simulink model "irep_force_control_simu"  (Simulink 8.5)
settings: Solver=ode3  StartTime=0.0  StopTime=inf  FixedStep=dt  RelTol=1e-3
InitFcn:
  | IREP_DEPENDENCY
  | init_omni
  | init_filters
  | init_invivo
  | init_telemanipulation
  | init_parker_xyz
  | init_magnetic_tracker
  | init_loadcell
  | init_scopes
  | init_homing
  | init_force_control
  | init_xpc_invivo_simu
undefined symbols (not defined in the file): ang_vel_scale, B_simu, beta, camera_home_voltage, counter_offset, dt, dt_trakstar, E_Y, encoder_counts, epsilon_robust_inverse, gear_ratio, HomingFineEps, HomingRoughEps, HomingRoughVelocity, I1_primary, I1_secondary, I2_primary, I2_secondary, irep_parameters_left, irep_parameters_right, joystick_filter_coeffs, K_d, K_i, K_naive_inv, K_p, k_right, L1l, L1r, L2l, L2r, L_zeus, left_arm_home_voltage, left_x0_parallelogram, LeftArmHomingDirectionVector, LeftArmHomingIntGain, lin_vel_scale, LOADCELL_BIAS, LOADCELL_GAIN, max_conf_space_speed, N_joystick, N_pots, N_trakstar, OmegaMax, OmegaMin, orientation_epsilon, position_epsilon, pots_filter_coeffs, q_eps_backlash, quadrature_mode, r, right_arm_home_voltage, RightArmHomingDirectionVector, RightArmHomingIntGain, screw_pitch, statics_param, tau_compression_bias, tau_compression_gains, tau_neutral_deadband, tau_tension_bias, tau_tension_gains ... (+14)
libraries: slrtlib x38, xpcrtudplib x13, xpcobsoletelib x13, simulink x6, dspswit3 x2, dspsigops x1
(part 4 of 6)

== system irep_force_control_simu/Trajectory Planner/Left Arm/High Level/Actuation Compensation/Parallelogram Backlash  Compensatior ==
  q des : Inport
  Backlash Compensator : MATLAB Function  TreatAsAtomicUnit=on
  Bus Selector : BusSelector  OutputSignals=q2; q3
  Discrete Derivative : simulink/Discrete/Discrete Derivative  gainval=1.0  ICPrevScaledInput=0.0  InputProcessing=Inherited  OutMin=[]  OutMax=[]  OutDataType=fixdt(1, 16)  OutScaling=2^-10  DoSatur=off
  comp close : Constant  Value=0.5
  comp open : Constant  Value=-1
  epsilon : Outport
  wires:
  q des/1 -> Bus Selector/1
  Bus Selector/1 -> Discrete Derivative/1, Backlash Compensator/1(q_curr)  "<q2; q3>"
  Discrete Derivative/1 -> Backlash Compensator/2(q_dot_curr)  "q dot curr"
  Backlash Compensator/1(epsilon) -> epsilon/1
  comp open/1 -> Backlash Compensator/3(q2_comp_open)
  comp close/1 -> Backlash Compensator/4(q2_comp_close)

== system irep_force_control_simu/Trajectory Planner/Left Arm/High Level/Configuration Space/Parallelogram ==
  Enable : EnablePort
  5th Order Polynomial : Subsystem
  b_des : Constant  Value=[left_x0_parallelogram z0_parallelogram]  SampleTime=dt
  b1 : Outport
  wires:
  5th Order Polynomial/1(b) -> b1/1
  b_des/1 -> 5th Order Polynomial/1(b des)

== system irep_force_control_simu/Trajectory Planner/Left Arm/High Level/Configuration Space/Stem ==
  Enable : EnablePort
  5th Order Polynomial : Subsystem
  Terminator : Terminator
  enable : Constant  Value=0  SampleTime=dt
  psi des : Constant  Value=[pi/2;0;pi/2;0;0]  SampleTime=dt
  psi0 : Constant  Value=[pi/2;0;pi/2;0;0]  SampleTime=dt
  psi dot : Outport  InitialOutput=zeros(5,1)
  wires:
  enable/1 -> 5th Order Polynomial/3(enable)
  psi0/1 -> 5th Order Polynomial/2(psi0)
  psi des/1 -> 5th Order Polynomial/1(psi des)
  5th Order Polynomial/2(psi dot) -> psi dot/1
  5th Order Polynomial/1(psi) -> Terminator/1

== system irep_force_control_simu/Trajectory Planner/Left Arm/High Level/Inverse Istantaneous Kinematics/Coordination Module ==
  b1 : Inport
  q par : Inport  Port=2
  5-Bar Inverse Kinematics : MATLAB Function  TreatAsAtomicUnit=on
  Add : Sum  Inputs=+-  SampleTime=dt
  Coordination Block : MATLAB Function  TreatAsAtomicUnit=on
  L0 : Constant  Value=L_zeus  SampleTime=dt
  b0 : Constant  Value=[x0_parallelogram z0_parallelogram]  SampleTime=dt
  q1 : Outport
  "q2, q3" : Outport  Port=2
  wires:
  Add/1 -> "q2, q3"/1
  q par/1 -> Coordination Block/2(q_par)
  b1/1 -> Coordination Block/1(b1)
  Coordination Block/1(q1) -> q1/1
  5-Bar Inverse Kinematics/1(q) -> Add/2
  L0/1 -> Coordination Block/3(L0)
  b0/1 -> 5-Bar Inverse Kinematics/1(b1)
  Coordination Block/2(q23) -> Add/1

== system irep_force_control_simu/Trajectory Planner/Left Arm/High Level/Inverse Istantaneous Kinematics/Jaw Open/Close Module ==
  note: Temp fix,
      | teleop GP not working
  sensors : Inport
  Enable : EnablePort
  Bus Selector : BusSelector  OutputSignals=MSG_Type,gripper
  Jaw Open/Close : MATLAB Function  TreatAsAtomicUnit=on
  MTML_GP_max : Constant
  MTML_GP_min : Constant  Value=-1.3
  Unit Delay : UnitDelay  SampleTime=-1
  q9 : Outport
  wires:
  sensors/1 -> Bus Selector/1
  Jaw Open/Close/1(y) -> q9/1, Unit Delay/1
  MTML_GP_max/1 -> Jaw Open/Close/3(MTM_GP_max)
  MTML_GP_min/1 -> Jaw Open/Close/4(MTM_GP_min)
  Bus Selector/2 -> Jaw Open/Close/2(u)  "<gripper>"
  Bus Selector/1 -> Jaw Open/Close/1(MSG_valid)  "<MSG_Type>"
  Unit Delay/1 -> Jaw Open/Close/5(q9_prev)

== system irep_force_control_simu/Trajectory Planner/Left Arm/High Level/Task Space/Compute Weigths ==
  sensors : Inport
  conf space : Inport  Port=2
  Bus Selector : BusSelector  OutputSignals=b1 curr,psi curr
  Bus Selector1 : BusSelector  OutputSignals=foot switches
  joint limits : Constant  Value=[-x0_parallelogram_max -x0_parallelogram z0_parallelogram z0_parallelogram_max theta_min1 theta_max theta_min2 theta_max wrist_min wrist_max]  SampleTime=dt
  select weights : MATLAB Function  TreatAsAtomicUnit=on
  w min : Constant  Value=w_min  SampleTime=dt
  weights : Outport
  wires:
  joint limits/1 -> select weights/3(joint_limits)
  Bus Selector/1 -> select weights/1(b1)  "<b1 curr>"
  Bus Selector/2 -> select weights/2(psi)  "<psi curr>"
  conf space/1 -> Bus Selector/1
  select weights/1(W) -> weights/1
  w min/1 -> select weights/4(w_min)
  sensors/1 -> Bus Selector1/1
  Bus Selector1/1 -> select weights/5(foot_switches)  "<foot switches>"

== system irep_force_control_simu/Trajectory Planner/Left Arm/High Level/Task Space/Desired Twist Module ==
  note: Desired Twist Module v 1.1 - © 2011 Andrea Bajo, Nabil Simaan
  current pose : Inport
  des pose : Inport  Port=2
  Bus Selector1 : BusSelector  OutputSignals=p in world,R in world
  Bus Selector2 : BusSelector  OutputSignals=position,R,MSG_Type
  Compute Twist : MATLAB Function  TreatAsAtomicUnit=on
  Omega Max : Constant  Value=OmegaMax  SampleTime=dt
  Omega Min : Constant  Value=OmegaMin  SampleTime=dt
  Terminator : Terminator
  V Max : Constant  Value=Vmax  SampleTime=dt
  V Min : Constant  Value=Vmin  SampleTime=dt
  ang vel scale : Constant  Value=ang_vel_scale  SampleTime=dt
  lin vel scale : Constant  Value=lin_vel_scale  SampleTime=dt
  orientation epsilon : Constant  Value=orientation_epsilon  SampleTime=dt
  position epsilon : Constant  Value=position_epsilon  SampleTime=dt
  x des : Outport
  wires:
  Bus Selector1/1 -> Compute Twist/4(p_curr)  "<p in world>"
  Compute Twist/1(x_des) -> x des/1
  current pose/1 -> Bus Selector1/1
  Bus Selector1/2 -> Compute Twist/5(R_curr)  "<R in world>"
  Bus Selector2/1 -> Compute Twist/1(p_des)  "<position>"
  Bus Selector2/2 -> Compute Twist/2(R_des)  "<R>"
  des pose/1 -> Bus Selector2/1
  Bus Selector2/3 -> Compute Twist/3(MSG_Type)  "<MSG_Type>"
  V Max/1 -> Compute Twist/6(Vmax)
  Omega Max/1 -> Compute Twist/10(OmegaMax)
  V Min/1 -> Compute Twist/7(Vmin)
  Omega Min/1 -> Compute Twist/11(OmegaMin)
  position epsilon/1 -> Compute Twist/8(position_epsilon)
  orientation epsilon/1 -> Compute Twist/12(orientation_epsilon)
  lin vel scale/1 -> Compute Twist/9(lin_vel_scale)
  ang vel scale/1 -> Compute Twist/13(ang_vel_scale)
  Compute Twist/2(theta) -> Terminator/1

== system irep_force_control_simu/Trajectory Planner/Left Arm/High Level/Task Space/Direct Kinematics IREP ==
  "b1, psi" : Inport
  Bus Creator : BusCreator  Inputs=2
  Bus Selector : BusSelector  OutputSignals=Parker insertion stage,b1 curr,psi curr
  Direct Kinematic IREP : MATLAB Function  TreatAsAtomicUnit=on
  IREP parameters : Constant  Value=irep_parameters_left  SampleTime=dt
  Current Pose : Outport
  wires:
  "b1, psi"/1 -> Bus Selector/1
  Bus Selector/2 -> Direct Kinematic IREP/2(b1)  "<b1 curr>"
  Bus Selector/3 -> Direct Kinematic IREP/3(psi)  "<psi curr>"
  Direct Kinematic IREP/1(p) -> Bus Creator/1  "p in world"
  Direct Kinematic IREP/2(R) -> Bus Creator/2  "R in world"
  Bus Creator/1 -> Current Pose/1
  IREP parameters/1 -> Direct Kinematic IREP/4(parameters)
  Bus Selector/1 -> Direct Kinematic IREP/1(b0)  "<Parker insertion stage>"

== system irep_force_control_simu/Trajectory Planner/Left Arm/High Level/Task Space/Jxpsi Inverse IREP ==
  x des : Inport
  weights : Inport  Port=2
  "b1, psi" : Inport  Port=3
  Bus Selector1 : BusSelector  OutputSignals=Parker insertion stage,b1 curr,psi curr
  IREP parameters : Constant  Value=irep_parameters_left  SampleTime=dt
  Jxpsi Inverse IREP : MATLAB Function  TreatAsAtomicUnit=on
  epsilon : Constant  Value=epsilon_robust_inverse  SampleTime=dt
  max conf space speed : Constant  Value=max_conf_space_speed  SampleTime=dt
  conf dot des : Outport  PortDimensions=8
  wires:
  x des/1 -> Jxpsi Inverse IREP/1(x_des)
  Bus Selector1/3 -> Jxpsi Inverse IREP/4(psi)  "<psi curr>"
  Bus Selector1/2 -> Jxpsi Inverse IREP/3(b1)  "<b1 curr>"
  "b1, psi"/1 -> Bus Selector1/1
  Jxpsi Inverse IREP/1(conf_space_dot) -> conf dot des/1
  epsilon/1 -> Jxpsi Inverse IREP/7(epsilon_in)
  Bus Selector1/1 -> Jxpsi Inverse IREP/2(b0)  "<Parker insertion stage>"
  max conf space speed/1 -> Jxpsi Inverse IREP/8(max_ang_speed)
  weights/1 -> Jxpsi Inverse IREP/6(weights)
  IREP parameters/1 -> Jxpsi Inverse IREP/5(parameters)

== system irep_force_control_simu/Trajectory Planner/Left Arm/High Level/Task Space/Receive Desired Pose from MTM ==
  note: Telemanipulation Module v 1.0 - © COPYRIGHT 2010 Andrea Bajo, Nabil Simaan
  Master : Inport
  Bus Creator : BusCreator
  Bus Selector : BusSelector  OutputSignals=position,orientation (quat),MSG_Type,gripper
  Quaternion To Rotation : MATLAB Function  TreatAsAtomicUnit=on
  "pose, flags" : Outport
  wires:
  Bus Creator/1 -> "pose, flags"/1
  Master/1 -> Bus Selector/1
  Bus Selector/1 -> Bus Creator/1  "<position>"
  Quaternion To Rotation/1(R) -> Bus Creator/2
  Bus Selector/2 -> Quaternion To Rotation/1(quat)  "<orientation (quat)>"
  Bus Selector/3 -> Bus Creator/3  "<MSG_Type>"
  Bus Selector/4 -> Bus Creator/4  "<gripper>"

== system irep_force_control_simu/Trajectory Planner/Left Arm/High Level/Task Space/right task space scope ==
  In : Inport
  Bus Selector7 : BusSelector  OutputSignals=position,R,gripper,MSG_Type
  Gain : Gain
  Mux : Mux  Inputs=5
  R_to_axis_angle1 : MATLAB Function  TreatAsAtomicUnit=on
  left task space : slrtlib/Displays and Logging/Scope   scopeno=18  scopetype=Host  autostart=on  viewmode=Numerical  formatstr=scope_format_left_task_space_des  grid=on  ylimits=[0,0]  nosamples=10  noprepostsamples=0  interleave=1  triggermode=FreeRun  triggersignal=1  trigsignalfromport=off  triggerlevel=0.0  triggerslope=Either  triggerscope=1  triggersample=0  filename=weights1.dat  mode=Lazy  writesize=512  autorestart=off  dynamicfilemode=off  maxwritefilesize=512*1024^2
  wires:
  Mux/1 -> Gain/1
  In/1 -> Bus Selector7/1
  Bus Selector7/2 -> R_to_axis_angle1/1(R)  "<R>"
  Gain/1 -> left task space/1
  Bus Selector7/1 -> Mux/1  "<position>"
  R_to_axis_angle1/1(n_vec) -> Mux/2
  R_to_axis_angle1/2(theta) -> Mux/3
  Bus Selector7/3 -> Mux/4  "<gripper>"
  Bus Selector7/4 -> Mux/5  "<MSG_Type>"

== system irep_force_control_simu/Trajectory Planner/Left Arm/Low Level/Home Procedure/Fine Homing - Integral Control ==
  error : Inport
  Enable : EnablePort  StatesWhenEnabling=reset
  Discrete-Time Integrator : DiscreteIntegrator  SampleTime=dt  LimitOutput=on  UpperSaturationLimit=8  LowerSaturationLimit=-8
  Integral Gain : Gain  Gain=diag(LeftArmHomingIntGain)  Multiplication=Matrix(K*u)  SampleTime=dt
  q_des_fine : Outport  InitialOutput=zeros(9,1)
  wires:
  error/1 -> Integral Gain/1
  Discrete-Time Integrator/1 -> q_des_fine/1
  Integral Gain/1 -> Discrete-Time Integrator/1

== system irep_force_control_simu/Trajectory Planner/Left Arm/Low Level/Home Procedure/Homing Flags ==
  u : Inport
  Homing Completion : MATLAB Function  TreatAsAtomicUnit=on
  HomingFineEps : Constant  Value=HomingFineEps  SampleTime=dt
  Terminator1 : Terminator
  Unit Delay : UnitDelay  InitialCondition=zeros(9,1)  SampleTime=-1
  dt : Constant  Value=dt  SampleTime=dt
  wires:
  Homing Completion/1(Homed) -> Terminator1/1
  HomingFineEps/1 -> Homing Completion/2(EPS)
  u/1 -> Homing Completion/1(u)
  Homing Completion/2(Homed_T) -> Unit Delay/1
  Unit Delay/1 -> Homing Completion/4(Homed_T_prev)
  dt/1 -> Homing Completion/3(dt)

== system irep_force_control_simu/Trajectory Planner/Right Arm/High Level/Actuation Compensation/Compute Taus ==
  In1 : Inport
  In2 : Inport  Port=2
  Compute Tau : MATLAB Function  TreatAsAtomicUnit=on
  k_right : Constant  Value=k_right  SampleTime=dt
  tau : Outport
  wires:
  k_right/1 -> Compute Tau/3(k_right)
  In1/1 -> Compute Tau/1(GradU)
  Compute Tau/1(tau) -> tau/1
  In2/1 -> Compute Tau/2(conf_space)

== system irep_force_control_simu/Trajectory Planner/Right Arm/High Level/Actuation Compensation/Grad U1 ==
  conf space : Inport
  q : Inport  Port=2
  Compute grad U : MATLAB Function  TreatAsAtomicUnit=on
  Constant : Constant  Value=L1r  SampleTime=dt
  E_Y : Constant  Value=E_Y  SampleTime=dt
  Ip : Constant  Value=I1_primary+I2_primary  SampleTime=dt
  Is : Constant  Value=I1_secondary+I2_secondary  SampleTime=dt
  beta : Constant  Value=beta  SampleTime=dt
  r : Constant  Value=r  SampleTime=dt
  theta_0 : Constant  Value=theta0  SampleTime=dt
  grad_U : Outport
  wires:
  Constant/1 -> Compute grad U/3(L_p)
  beta/1 -> Compute grad U/9(beta)
  theta_0/1 -> Compute grad U/8(theta_0)
  r/1 -> Compute grad U/4(r)
  Ip/1 -> Compute grad U/6(Ip)
  E_Y/1 -> Compute grad U/5(E_Y)
  Compute grad U/1(grad_U) -> grad_U/1
  conf space/1 -> Compute grad U/1(conf_space)
  q/1 -> Compute grad U/2(q)
  Is/1 -> Compute grad U/7(Is)

== system irep_force_control_simu/Trajectory Planner/Right Arm/High Level/Actuation Compensation/Grad U2 ==
  conf space : Inport
  q : Inport  Port=2
  Compute grad U : MATLAB Function  TreatAsAtomicUnit=on
  Constant : Constant  Value=L2r  SampleTime=dt
  E_Y : Constant  Value=E_Y  SampleTime=dt
  Ip : Constant  Value=I2_primary  SampleTime=dt
  Is : Constant  Value=I2_secondary  SampleTime=dt
  beta : Constant  Value=beta  SampleTime=dt
  r : Constant  Value=r  SampleTime=dt
  theta_0 : Constant  Value=theta0  SampleTime=dt
  grad_U : Outport
  wires:
  Is/1 -> Compute grad U/7(Is)
  q/1 -> Compute grad U/2(q)
  conf space/1 -> Compute grad U/1(conf_space)
  Compute grad U/1(grad_U) -> grad_U/1
  E_Y/1 -> Compute grad U/5(E_Y)
  Ip/1 -> Compute grad U/6(Ip)
  r/1 -> Compute grad U/4(r)
  theta_0/1 -> Compute grad U/8(theta_0)
  beta/1 -> Compute grad U/9(beta)
  Constant/1 -> Compute grad U/3(L_p)

== system irep_force_control_simu/Trajectory Planner/Right Arm/High Level/Actuation Compensation/Parallelogram Backlash  Compensatior ==
  q des : Inport
  Backlash Compensator : MATLAB Function  TreatAsAtomicUnit=on
  Bus Selector : BusSelector  OutputSignals=q2;q3
  Discrete Derivative : simulink/Discrete/Discrete Derivative  gainval=1.0  ICPrevScaledInput=0.0  InputProcessing=Inherited  OutMin=[]  OutMax=[]  OutDataType=fixdt(1, 16)  OutScaling=2^-10  DoSatur=off
  comp close : Constant  Value=0
  comp close1 : Constant  Value=0.6
  comp open : Constant  Value=0
  comp open1 : Constant  Value=-1.2
  epsilon : Outport
  wires:
  q des/1 -> Bus Selector/1
  Bus Selector/1 -> Discrete Derivative/1, Backlash Compensator/1(q_curr)  "<q2;q3>"
  Discrete Derivative/1 -> Backlash Compensator/2(q_dot_curr)  "q dot curr"
  Backlash Compensator/1(epsilon) -> epsilon/1
  comp open/1 -> Backlash Compensator/3(q1_comp_open)
  comp close/1 -> Backlash Compensator/4(q1_comp_close)
  comp open1/1 -> Backlash Compensator/5(q2_comp_open)
  comp close1/1 -> Backlash Compensator/6(q2_comp_close)

== system irep_force_control_simu/Trajectory Planner/Right Arm/High Level/Actuation Compensation/get q_dot sign ==
  conf_space_dot : Inport
  conf_space : Inport  Port=2
  Dead Zone : DeadZone  LowerValue=-1e-3  UpperValue=1e-3  SaturateOnIntegerOverflow=on
  Unit Delay : UnitDelay  SampleTime=-1
  compute q_dot : MATLAB Function  TreatAsAtomicUnit=on
  q_dot_sign : MATLAB Function  TreatAsAtomicUnit=on
  q_dot_sgn : Outport
  wires:
  conf_space_dot/1 -> compute q_dot/2(conf_space_dot)
  conf_space/1 -> compute q_dot/1(conf_space)
  q_dot_sign/1(q_dot_sign_out) -> q_dot_sgn/1, Unit Delay/1
  Unit Delay/1 -> q_dot_sign/2(q_dot_sign_prev)
  compute q_dot/1(q_dot) -> Dead Zone/1
  Dead Zone/1 -> q_dot_sign/1(q_dot_sign_in)

== system irep_force_control_simu/Trajectory Planner/Right Arm/High Level/Actuation Compensation/q_eps 5th order poly ==
  q_eps_ref : Inport
  enable : Inport  Port=2
  Constant : Constant  Value=q_eps_backlash
  Digital Clock : DigitalClock  SampleTime=dt
  Embedded MATLAB Function : MATLAB Function  TreatAsAtomicUnit=on
  Terminator : Terminator
  Unit Delay : UnitDelay  SampleTime=dt
  Unit Delay1 : UnitDelay  SampleTime=dt
  Unit Delay2 : UnitDelay  InitialCondition=zeros(9,1)  SampleTime=dt
  tf : Constant  Value=5  SampleTime=dt
  q_eps_des : Outport
  wires:
  Embedded MATLAB Function/3(confn) -> Unit Delay/1
  Unit Delay/1 -> Embedded MATLAB Function/5(conf)
  Embedded MATLAB Function/4(t0n) -> Unit Delay1/1
  Embedded MATLAB Function/5(p0n) -> Unit Delay2/1
  Unit Delay2/1 -> Embedded MATLAB Function/7(p0)
  Unit Delay1/1 -> Embedded MATLAB Function/6(t0)
  Digital Clock/1 -> Embedded MATLAB Function/4(tc)
  q_eps_ref/1 -> Embedded MATLAB Function/1(p_des)
  Embedded MATLAB Function/1(p) -> q_eps_des/1
  tf/1 -> Embedded MATLAB Function/3(tf)
  enable/1 -> Embedded MATLAB Function/8(enable)
  Constant/1 -> Embedded MATLAB Function/2(p_curr)
  Embedded MATLAB Function/2(pdot) -> Terminator/1

== system irep_force_control_simu/Trajectory Planner/Right Arm/High Level/Configuration Space/Parallelogram ==
  Enable : EnablePort
  5th Order Polynomial : Subsystem
  b_des : Constant  Value=[x0_parallelogram z0_parallelogram]  SampleTime=dt
  b1 : Outport
  wires:
  b_des/1 -> 5th Order Polynomial/1(b des)
  5th Order Polynomial/1(b) -> b1/1

== system irep_force_control_simu/Trajectory Planner/Right Arm/High Level/Configuration Space/Stem ==
  Enable : EnablePort
  5th Order Polynomial : Subsystem
  Terminator : Terminator
  enable : Constant  Value=0  SampleTime=dt
  psi des : Constant  Value=[pi/2;0;pi/2;0;0]  SampleTime=dt
  psi0 : Constant  Value=[pi/2;0;pi/2;0;0]  SampleTime=dt
  psi dot : Outport  InitialOutput=zeros(5,1)
  wires:
  5th Order Polynomial/2(psi dot) -> psi dot/1
  psi des/1 -> 5th Order Polynomial/1(psi des)
  psi0/1 -> 5th Order Polynomial/2(psi0)
  enable/1 -> 5th Order Polynomial/3(enable)
  5th Order Polynomial/1(psi) -> Terminator/1

== system irep_force_control_simu/Trajectory Planner/Right Arm/High Level/Inverse Istantaneous Kinematics/Coordination Module ==
  b1 : Inport
  q par : Inport  Port=2
  5-Bar Inverse Kinematics : MATLAB Function  TreatAsAtomicUnit=on
  Add : Sum  Inputs=+-  SampleTime=dt
  Coordination Block : MATLAB Function  TreatAsAtomicUnit=on
  L0 : Constant  Value=L_zeus  SampleTime=dt
  b0 : Constant  Value=[x0_parallelogram z0_parallelogram]  SampleTime=dt
  q1 : Outport
  "q2, q3" : Outport  Port=2
  wires:
  Add/1 -> "q2, q3"/1
  q par/1 -> Coordination Block/2(q_par)
  b1/1 -> Coordination Block/1(b1)
  Coordination Block/1(q1) -> q1/1
  5-Bar Inverse Kinematics/1(q) -> Add/2
  L0/1 -> Coordination Block/3(L0)
  b0/1 -> 5-Bar Inverse Kinematics/1(b1)
  Coordination Block/2(q23) -> Add/1

== system irep_force_control_simu/Trajectory Planner/Right Arm/High Level/Inverse Istantaneous Kinematics/Jaw Open/Close Module ==
  sensors : Inport
  Enable : EnablePort
  Bus Selector : BusSelector  OutputSignals=MSG_Type,gripper
  Jaw Open/Close : MATLAB Function  TreatAsAtomicUnit=on
  MTM_GP_max : Constant  Value=1.05
  MTM_GP_min : Constant  Value=-0.48
  Unit Delay : UnitDelay  SampleTime=-1
  Unit Delay1 : UnitDelay  SampleTime=-1
  q9 : Outport
  wires:
  sensors/1 -> Bus Selector/1
  Jaw Open/Close/1(y) -> Unit Delay/1, Unit Delay1/1
  Bus Selector/2 -> Jaw Open/Close/2(u)  "<gripper>"
  MTM_GP_max/1 -> Jaw Open/Close/3(MTM_GP_max)
  MTM_GP_min/1 -> Jaw Open/Close/4(MTM_GP_min)
  Bus Selector/1 -> Jaw Open/Close/1(MSG_valid)  "<MSG_Type>"
  Unit Delay/1 -> Jaw Open/Close/5(q9_prev)
  Unit Delay1/1 -> q9/1

== system irep_force_control_simu/Trajectory Planner/Right Arm/High Level/Task Space/Compute Weigths ==
  sensors : Inport
  conf space : Inport  Port=2
  Bus Selector : BusSelector  OutputSignals=b1 curr,psi curr
  Bus Selector1 : BusSelector  OutputSignals=foot switches
  joint limits : Constant  Value=[x0_parallelogram x0_parallelogram_max z0_parallelogram z0_parallelogram_max theta_min1 theta_max theta_min2 theta_max wrist_min wrist_max]  SampleTime=dt
  select weights : MATLAB Function  TreatAsAtomicUnit=on
  w_min : Constant  Value=w_min  SampleTime=dt
  weights : Outport
  wires:
  joint limits/1 -> select weights/3(joint_limits)
  Bus Selector/1 -> select weights/1(b1)  "<b1 curr>"
  Bus Selector/2 -> select weights/2(psi)  "<psi curr>"
  conf space/1 -> Bus Selector/1
  select weights/1(W) -> weights/1
  w_min/1 -> select weights/4(w_min)
  sensors/1 -> Bus Selector1/1
  Bus Selector1/1 -> select weights/5(foot_switches)  "<foot switches>"

== system irep_force_control_simu/Trajectory Planner/Right Arm/High Level/Task Space/Desired Twist Module ==
  note: Desired Twist Module v 1.1 - © 2011 Andrea Bajo, Nabil Simaan
  current pose : Inport
  des pose : Inport  Port=2
  Bus Selector1 : BusSelector  OutputSignals=p in world,R in world
  Bus Selector2 : BusSelector  OutputSignals=position,R,MSG_Type
  Compute Twist : MATLAB Function  TreatAsAtomicUnit=on
  Omega Max : Constant  Value=OmegaMax  SampleTime=dt
  Omega Min : Constant  Value=OmegaMin  SampleTime=dt
  V Max : Constant  Value=Vmax  SampleTime=dt
  V Min : Constant  Value=Vmin  SampleTime=dt
  ang vel scale : Constant  Value=ang_vel_scale  SampleTime=dt
  lin vel scale : Constant  Value=lin_vel_scale  SampleTime=dt
  orientation epsilon : Constant  Value=orientation_epsilon  SampleTime=dt
  position epsilon : Constant  Value=position_epsilon  SampleTime=dt
  x des : Outport
  wires:
  Bus Selector1/1 -> Compute Twist/4(p_curr)  "<p in world>"
  Compute Twist/1(x_des) -> x des/1
  current pose/1 -> Bus Selector1/1
  Bus Selector1/2 -> Compute Twist/5(R_curr)  "<R in world>"
  Bus Selector2/1 -> Compute Twist/1(p_des)  "<position>"
  Bus Selector2/2 -> Compute Twist/2(R_des)  "<R>"
  des pose/1 -> Bus Selector2/1
  Bus Selector2/3 -> Compute Twist/3(MSG_Type)  "<MSG_Type>"
  V Max/1 -> Compute Twist/6(Vmax)
  Omega Max/1 -> Compute Twist/10(OmegaMax)
  V Min/1 -> Compute Twist/7(Vmin)
  Omega Min/1 -> Compute Twist/11(OmegaMin)
  position epsilon/1 -> Compute Twist/8(position_epsilon)
  orientation epsilon/1 -> Compute Twist/12(orientation_epsilon)
  lin vel scale/1 -> Compute Twist/9(lin_vel_scale)
  ang vel scale/1 -> Compute Twist/13(ang_vel_scale)

== system irep_force_control_simu/Trajectory Planner/Right Arm/High Level/Task Space/Direct Kinematics IREP ==
  "b1, psi" : Inport
  Bus Creator : BusCreator  Inputs=2
  Bus Selector : BusSelector  OutputSignals=Parker insertion stage,b1 curr,psi curr
  Direct Kinematic IREP : MATLAB Function  TreatAsAtomicUnit=on
  IREP parameters : Constant  Value=irep_parameters_right  SampleTime=dt
  Current Pose : Outport
  wires:
  "b1, psi"/1 -> Bus Selector/1
  Bus Selector/2 -> Direct Kinematic IREP/2(b1)  "<b1 curr>"
  Bus Selector/3 -> Direct Kinematic IREP/3(psi)  "<psi curr>"
  Direct Kinematic IREP/1(p) -> Bus Creator/1  "p in world"
  Direct Kinematic IREP/2(R) -> Bus Creator/2  "R in world"
  Bus Creator/1 -> Current Pose/1
  IREP parameters/1 -> Direct Kinematic IREP/4(parameters)
  Bus Selector/1 -> Direct Kinematic IREP/1(b0)  "<Parker insertion stage>"

== system irep_force_control_simu/Trajectory Planner/Right Arm/High Level/Task Space/Jxpsi Inverse IREP ==
  x des : Inport
  weights : Inport  Port=2
  "b1, psi" : Inport  Port=3
  Bus Selector : BusSelector  OutputSignals=Parker insertion stage,b1 curr,psi curr
  IREP parameters : Constant  Value=irep_parameters_right  SampleTime=dt
  Jxpsi Inverse IREP : MATLAB Function  TreatAsAtomicUnit=on
  epsilon : Constant  Value=epsilon_robust_inverse  SampleTime=dt
  max conf space speed : Constant  Value=max_conf_space_speed  SampleTime=dt
  conf dot des : Outport  PortDimensions=[8 1]
  wires:
  IREP parameters/1 -> Jxpsi Inverse IREP/5(parameters)
  x des/1 -> Jxpsi Inverse IREP/1(x_des)
  Bus Selector/3 -> Jxpsi Inverse IREP/4(psi)  "<psi curr>"
  Bus Selector/2 -> Jxpsi Inverse IREP/3(b1)  "<b1 curr>"
  "b1, psi"/1 -> Bus Selector/1
  Jxpsi Inverse IREP/1(conf_space_dot) -> conf dot des/1
  epsilon/1 -> Jxpsi Inverse IREP/7(epsilon_in)
  weights/1 -> Jxpsi Inverse IREP/6(weights)
  Bus Selector/1 -> Jxpsi Inverse IREP/2(b0)  "<Parker insertion stage>"
  max conf space speed/1 -> Jxpsi Inverse IREP/8(max_ang_speed)

== system irep_force_control_simu/Trajectory Planner/Right Arm/High Level/Task Space/Receive Desired Pose from MTM ==
  note: Telemanipulation Module v 1.0 - © COPYRIGHT 2010 Andrea Bajo, Nabil Simaan
  Master : Inport
  Bus Creator : BusCreator
  Bus Selector : BusSelector  OutputSignals=position,orientation (quat),MSG_Type,gripper
  Quaternion To Rotation : MATLAB Function  TreatAsAtomicUnit=on
  "pose, flags" : Outport
  wires:
  Bus Creator/1 -> "pose, flags"/1
  Master/1 -> Bus Selector/1
  Bus Selector/1 -> Bus Creator/1  "<position>"
  Quaternion To Rotation/1(R) -> Bus Creator/2
  Bus Selector/2 -> Quaternion To Rotation/1(quat)  "<orientation (quat)>"
  Bus Selector/3 -> Bus Creator/3  "<MSG_Type>"
  Bus Selector/4 -> Bus Creator/4  "<gripper>"

== system irep_force_control_simu/Trajectory Planner/Right Arm/High Level/Task Space/right task space scope ==
  des : Inport
  Bus Selector7 : BusSelector  OutputSignals=position,R,gripper,MSG_Type
  Gain : Gain
  Mux : Mux  Inputs=5
  R_to_axis_angle1 : MATLAB Function  TreatAsAtomicUnit=on
  right task space : slrtlib/Displays and Logging/Scope   scopeno=26  scopetype=Host  autostart=on  viewmode=Numerical  formatstr=scope_format_right_task_space_des  grid=on  ylimits=[0,0]  nosamples=10  noprepostsamples=0  interleave=1  triggermode=FreeRun  triggersignal=1  trigsignalfromport=off  triggerlevel=0.0  triggerslope=Either  triggerscope=1  triggersample=0  filename=weights1.dat  mode=Lazy  writesize=512  autorestart=off  dynamicfilemode=off  maxwritefilesize=512*1024^2
  wires:
  Mux/1 -> Gain/1
  des/1 -> Bus Selector7/1
  Bus Selector7/2 -> R_to_axis_angle1/1(R)  "<R>"
  Gain/1 -> right task space/1
  Bus Selector7/3 -> Mux/4  "<gripper>"
  R_to_axis_angle1/1(n_vec) -> Mux/2
  R_to_axis_angle1/2(theta) -> Mux/3
  Bus Selector7/1 -> Mux/1  "<position>"
  Bus Selector7/4 -> Mux/5  "<MSG_Type>"

== system irep_force_control_simu/Trajectory Planner/Right Arm/Low Level/Home Procedure/Fine Homing - Integral Control ==
  error : Inport
  Enable : EnablePort  StatesWhenEnabling=reset
  Discrete-Time Integrator : DiscreteIntegrator  SampleTime=dt  LimitOutput=on  UpperSaturationLimit=8  LowerSaturationLimit=-8
  Integral Gain : Gain  Gain=diag(RightArmHomingIntGain)  Multiplication=Matrix(K*u)  SampleTime=dt
  q_des_fine : Outport  InitialOutput=zeros(9,1)
  wires:
  error/1 -> Integral Gain/1
  Discrete-Time Integrator/1 -> q_des_fine/1
  Integral Gain/1 -> Discrete-Time Integrator/1

== system irep_force_control_simu/Trajectory Planner/Left Arm/High Level/Configuration Space/Parallelogram/5th Order Polynomial ==
  b des : Inport
  Digital Clock : DigitalClock  SampleTime=dt
  Embedded MATLAB Function : MATLAB Function  TreatAsAtomicUnit=on
  Unit Delay : UnitDelay  SampleTime=dt
  Unit Delay1 : UnitDelay  SampleTime=dt
  Unit Delay2 : UnitDelay  InitialCondition=[left_x0_parallelogram;z0_parallelogram]  SampleTime=dt
  tf : Constant  Value=5  SampleTime=dt
  b : Outport
  wires:
  tf/1 -> Embedded MATLAB Function/2(tf)
  Embedded MATLAB Function/1(pd) -> b/1
  b des/1 -> Embedded MATLAB Function/1(p_des)
  Digital Clock/1 -> Embedded MATLAB Function/3(tc)
  Unit Delay1/1 -> Embedded MATLAB Function/5(t0)
  Unit Delay2/1 -> Embedded MATLAB Function/6(p0)
  Embedded MATLAB Function/4(p0n) -> Unit Delay2/1
  Embedded MATLAB Function/3(t0n) -> Unit Delay1/1
  Unit Delay/1 -> Embedded MATLAB Function/4(conf)
  Embedded MATLAB Function/2(confn) -> Unit Delay/1

== system irep_force_control_simu/Trajectory Planner/Left Arm/High Level/Configuration Space/Stem/5th Order Polynomial ==
  psi des : Inport
  psi0 : Inport  Port=2
  enable : Inport  Port=3
  Digital Clock : DigitalClock  SampleTime=dt
  Embedded MATLAB Function : MATLAB Function  TreatAsAtomicUnit=on
  Unit Delay : UnitDelay  SampleTime=dt
  Unit Delay1 : UnitDelay  SampleTime=dt
  Unit Delay2 : UnitDelay  InitialCondition=zeros(5,1)  SampleTime=dt
  tf : Constant  Value=5  SampleTime=dt
  psi : Outport
  psi dot : Outport  Port=2
  wires:
  Embedded MATLAB Function/2(pdot) -> psi dot/1
  psi0/1 -> Embedded MATLAB Function/2(p_curr)
  enable/1 -> Embedded MATLAB Function/8(enable)
  tf/1 -> Embedded MATLAB Function/3(tf)
  Embedded MATLAB Function/1(p) -> psi/1
  psi des/1 -> Embedded MATLAB Function/1(p_des)
  Digital Clock/1 -> Embedded MATLAB Function/4(tc)
  Unit Delay1/1 -> Embedded MATLAB Function/6(t0)
  Unit Delay2/1 -> Embedded MATLAB Function/7(p0)
  Embedded MATLAB Function/5(p0n) -> Unit Delay2/1
  Embedded MATLAB Function/4(t0n) -> Unit Delay1/1
  Unit Delay/1 -> Embedded MATLAB Function/5(conf)
  Embedded MATLAB Function/3(confn) -> Unit Delay/1

== system irep_force_control_simu/Trajectory Planner/Right Arm/High Level/Configuration Space/Parallelogram/5th Order Polynomial ==
  b des : Inport
  Digital Clock : DigitalClock  SampleTime=dt
  Embedded MATLAB Function : MATLAB Function  TreatAsAtomicUnit=on
  Unit Delay : UnitDelay  SampleTime=dt
  Unit Delay1 : UnitDelay  SampleTime=dt
  Unit Delay2 : UnitDelay  InitialCondition=[x0_parallelogram;z0_parallelogram]  SampleTime=dt
  tf : Constant  Value=5  SampleTime=dt
  b : Outport
  wires:
  Embedded MATLAB Function/2(confn) -> Unit Delay/1
  Unit Delay/1 -> Embedded MATLAB Function/4(conf)
  Embedded MATLAB Function/3(t0n) -> Unit Delay1/1
  Embedded MATLAB Function/4(p0n) -> Unit Delay2/1
  Unit Delay2/1 -> Embedded MATLAB Function/6(p0)
  Unit Delay1/1 -> Embedded MATLAB Function/5(t0)
  Digital Clock/1 -> Embedded MATLAB Function/3(tc)
  b des/1 -> Embedded MATLAB Function/1(p_des)
  Embedded MATLAB Function/1(pd) -> b/1
  tf/1 -> Embedded MATLAB Function/2(tf)

== system irep_force_control_simu/Trajectory Planner/Right Arm/High Level/Configuration Space/Stem/5th Order Polynomial ==
  psi des : Inport
  psi0 : Inport  Port=2
  enable : Inport  Port=3
  Digital Clock : DigitalClock  SampleTime=dt
  Embedded MATLAB Function : MATLAB Function  TreatAsAtomicUnit=on
  Unit Delay : UnitDelay  SampleTime=dt
  Unit Delay1 : UnitDelay  SampleTime=dt
  Unit Delay2 : UnitDelay  InitialCondition=zeros(5,1)  SampleTime=dt
  tf : Constant  Value=5  SampleTime=dt
  psi : Outport
  psi dot : Outport  Port=2
  wires:
  Embedded MATLAB Function/3(confn) -> Unit Delay/1
  Unit Delay/1 -> Embedded MATLAB Function/5(conf)
  Embedded MATLAB Function/4(t0n) -> Unit Delay1/1
  Embedded MATLAB Function/5(p0n) -> Unit Delay2/1
  Unit Delay2/1 -> Embedded MATLAB Function/7(p0)
  Unit Delay1/1 -> Embedded MATLAB Function/6(t0)
  Digital Clock/1 -> Embedded MATLAB Function/4(tc)
  psi des/1 -> Embedded MATLAB Function/1(p_des)
  Embedded MATLAB Function/1(p) -> psi/1
  tf/1 -> Embedded MATLAB Function/3(tf)
  enable/1 -> Embedded MATLAB Function/8(enable)
  psi0/1 -> Embedded MATLAB Function/2(p_curr)
  Embedded MATLAB Function/2(pdot) -> psi dot/1

== matlab function Trajectory Planner/Right Arm/High Level/Inverse Istantaneous Kinematics/Coordination Module/Coordination Block ==
  data: b1 input double; q1 output double; q_par input double; L0 input double; q23 output double
%--------------------------------------------------------------------------
%               Compute length of passive segment
%
%   Author: Andrea Bajo - andrea.bajo@vanderbilt.edu
%           Nabil Simaan - nabil.simaan@vanderbilt.edu
%
%           A.R.M.A. Lab
%           © 2010 Vanderbilt University
%
%   Created: 11:51 AM, October 22, 2010
%
%   Variables:
%       q1=q_ins+compensation insertion of the stem the passive stem.
%          q1=q_ins corresponds to straight stem configuration.
%       q_ins is the axial insertion of the passive stem (desired value).
%          q_ins=0 corresponds to the home position of the misumi slide.
%       q23 [q2;q3] is the desired postion of the parallelogram joints
%          with respect to straight configuration (right no b1 = [3.8;50.8])
%       b1=the desired position of the snake base=parallelogram tip in {B0}
%       {B0} is a right handed frame with z axis along center of IREP
%           stem and x axis pointing in the direction of parallelogram
%           opening
%       q_par=the corresponding q2, q3 values for the desired b1. 
%       L0=initial length of passive stem at home configuration. 
%       alpha is a compensation factor for accounting for the required pulling when the passive stem is commanded forward
%--------------------------------------------------------------------------
function [q1,q23]  = fcn(b1,q_par,L0)
%#eml

L = get_length_for_coordination(b1);
q_offset = L-L0;
q1 = q_offset;
q23 = q_par - [q_offset;q_offset];

== matlab function Trajectory Planner/Right Arm/High Level/Inverse Istantaneous Kinematics/5-Bar Inverse Kinematics ==
  data: b1 input double; q output double
function q  = fcn(b1)
%#eml
% if b1(1) > 3.8
%     x = b1(1)*1.6;
%     z = b1(2) - (b1(1)-3.8)/(20-3.8) * 6.5;
% else
    x = b1(1);
    z = b1(2);
% end
[q1 q2] = FiveBarInvKin(x,z);
q = [q1;q2];

== matlab function Trajectory Planner/RZ/Joystick Control for RZ/Embedded MATLAB Function ==
  data: u input double; y output double
function y = fcn(u)
%#eml

y = round(u*10)/10;

== matlab function Trajectory Planner/Right Arm/High Level/Task Space/Receive Desired Pose from MTM/Quaternion To Rotation ==
  data: quat input double; R output double
function R = fcn(quat)
%#eml
if norm(quat)==0
    quat = [1;0;0;0];
end
R = quat2rot(quat);

== matlab function Trajectory Planner/Right Arm/High Level/Configuration Space/Parallelogram/5th Order Polynomial/Embedded MATLAB Function ==
  data: p_des input double; tf input double; tc input double; pd output double; conf input double; confn output double; t0 input double; t0n output double; p0n output double; p0 input double
function [pd,confn,t0n,p0n] = fifth_order_p(p_des,tf,tc,conf,t0,p0)

% if enable == 0                  % Configuration space is not used (pdot = 0). 
%     p = p_curr;          % However we do want to record the current 
%     confn = 0;                  % position in order to be ready as soon 
%     t0n = tc;                   % as the enable becomes 1. 
%     p0n = p_curr;
% else
    if (p_des-p0)'*(p_des-p0) > 0
        if conf == 0                % conf = 0 means that the 5th order poly 
            p0n = p0;               % is not configured for the desired trajectory.
            t0n = tc;               % Therefore, the block is initialized.
            confn = 1;
            pd = zeros(2,1);
%              p = p0;
        else
            p0n = p0;
            t0n = t0;
            confn = conf;
            % 5th order polynomial
            a0 = p0;
            a4 = -15*(p_des-p0);
            a3 = -2/3 * a4;
            a5 = -2/5 * a4;
            t = tc-t0;
%             tau = t/tf;
            if t < tf
%                 p = a0 + a3 * tau^3 + a4 * tau^4 + a5 * tau^5;
                pd = 3*a3*t^2/tf^3 + 4*a4*t^3/tf^4 + 5*a5*t^4/tf^5;
            else
%                 p = p_des;
                pd = zeros(2,1);
                p0n = p_des;
            end
        end
    else
%         p = p_des;
        pd = zeros(2,1);
        confn = 0;
        p0n = p0;
        t0n = t0;
    end
% end
%------------------------------------------------------------------------

== matlab function Trajectory Planner/Right Arm/High Level/Inverse Istantaneous Kinematics/Coordination Module/5-Bar Inverse Kinematics ==
  data: b1 input double; q output double
function q  = fcn(b1)
%#eml
x = b1(1);
z = b1(2);
[q1 q2] = FiveBarInvKin(x,z);
q = [q1;q2];

== matlab function Trajectory Planner/Left Arm/High Level/Configuration Space/Parallelogram/5th Order Polynomial/Embedded MATLAB Function ==
  data: p_des input double; tf input double; tc input double; pd output double; conf input double; confn output double; t0 input double; t0n output double; p0n output double; p0 input double
function [pd,confn,t0n,p0n] = fifth_order_p(p_des,tf,tc,conf,t0,p0)

% if enable == 0                  % Configuration space is not used (pdot = 0). 
%     p = p_curr;          % However we do want to record the current 
%     confn = 0;                  % position in order to be ready as soon 
%     t0n = tc;                   % as the enable becomes 1. 
%     p0n = p_curr;
% else
    if (p_des-p0)'*(p_des-p0) > 0
        if conf == 0                % conf = 0 means that the 5th order poly 
            p0n = p0;               % is not configured for the desired trajectory.
            t0n = tc;               % Therefore, the block is initialized.
            confn = 1;
            pd = zeros(2,1);
%              p = p0;
        else
            p0n = p0;
            t0n = t0;
            confn = conf;
            % 5th order polynomial
            a0 = p0;
            a4 = -15*(p_des-p0);
            a3 = -2/3 * a4;
            a5 = -2/5 * a4;
            t = tc-t0;
%             tau = t/tf;
            if t < tf
%                 p = a0 + a3 * tau^3 + a4 * tau^4 + a5 * tau^5;
                pd = 3*a3*t^2/tf^3 + 4*a4*t^3/tf^4 + 5*a5*t^4/tf^5;
            else
%                 p = p_des;
                pd = zeros(2,1);
                p0n = p_des;
            end
        end
    else
%         p = p_des;
        pd = zeros(2,1);
        confn = 0;
        p0n = p0;
        t0n = t0;
    end
% end
%------------------------------------------------------------------------

== matlab function Trajectory Planner/Left Arm/High Level/Configuration Space/Stem/5th Order Polynomial/Embedded MATLAB Function ==
  data: p_des input double; p_curr input double; tf input double; tc input double; p output double; pdot output double; conf input double; confn output double; t0 input double; t0n output double; p0n output double; p0 input double; enable input double
function [p,pdot,confn,t0n,p0n] = fifth_order_p(p_des,p_curr,tf,tc,conf,t0,p0,enable)

if enable == 0                  % Configuration space is not used (pdot = 0). 
    p = p_curr;          % However we do want to record the current 
    confn = 0;                  % position in order to be ready as soon 
    t0n = tc;                   % as the enable becomes 1. 
    p0n = p_curr;
    pdot = zeros(5,1);
else
    if (p_des-p0)'*(p_des-p0) > 0
        if conf == 0                % conf = 0 means that the 5th order poly 
            p0n = p0;               % is not configured for the desired trajectory.
            t0n = tc;               % Therefore, the block is initialized.
            confn = 1;
            p = p0;
            pdot = zeros(5,1);
        else
            p0n = p0;
            t0n = t0;
            confn = conf;
            % 5th order polynomial
            a0 = p0;
            a4 = -15*(p_des-p0);
            a3 = -2/3 * a4;
            a5 = -2/5 * a4;
            t = tc-t0;
            tau = t/tf;
            if t < tf
                p = a0 + a3 * tau^3 + a4 * tau^4 + a5 * tau^5;
                pdot = 3*a3*t^2/tf^3 + 4*a4*t^3/tf^4 + 5*a5*t^4/tf^5;
            else
                p = p_des;
                pdot = zeros(5,1);
                p0n = p_des;
            end
        end
    else
        p = p_des;
        pdot = zeros(5,1);
        confn = 0;
        p0n = p0;
        t0n = t0;
    end
end
%------------------------------------------------------------------------

== matlab function Trajectory Planner/Camera/Homing Procedure/Homing Completion ==
  data: u input double; y output double
function y = fcn(u)
%#eml
y = zeros(3,1);
u = abs(u);
if u(1) <= 0.002
    y(1) = 1;
end
if u(2) <= 0.002
    y(2) = 1;
end
if u(3) <= 0.002
    y(3) = 1;
end

== matlab function Trajectory Planner/Left Arm/High Level/Inverse Istantaneous Kinematics/5-Bar Inverse Kinematics ==
  data: b1 input double; q output double
function q  = fcn(b1)
%#eml
b1 = [-b1(1);b1(2)];

x = b1(1);
z = b1(2);

[q1 q2] = FiveBarInvKin(x,z);
q = [q1;q2];

== matlab function Trajectory Planner/Left Arm/High Level/Inverse Istantaneous Kinematics/Coordination Module/5-Bar Inverse Kinematics ==
  data: b1 input double; q output double
function q  = fcn(b1)
%#eml
x = b1(1);
z = b1(2);
[q1 q2] = FiveBarInvKin(x,z);
q = [q1;q2];

== matlab function Trajectory Planner/Left Arm/High Level/Inverse Istantaneous Kinematics/Coordination Module/Coordination Block ==
  data: b1 input double; q1 output double; q_par input double; L0 input double; q23 output double
%--------------------------------------------------------------------------
%               Compute length of passive segment
%
%   Author: Andrea Bajo - andrea.bajo@vanderbilt.edu
%           Nabil Simaan - nabil.simaan@vanderbilt.edu
%
%           A.R.M.A. Lab
%           © 2010 Vanderbilt University
%
%   Created: 11:51 AM, October 22, 2010
%
%   Variables:
%       q1=q_ins+compensation insertion of the stem the passive stem.
%          q1=q_ins corresponds to straight stem configuration.
%       q_ins is the axial insertion of the passive stem (desired value).
%          q_ins=0 corresponds to the home position of the misumi slide.
%       q23 [q2;q3] is the desired postion of the parallelogram joints
%          with respect to straight configuration (right no b1 = [3.8;50.8])
%       b1=the desired position of the snake base=parallelogram tip in {B0}
%       {B0} is a right handed frame with z axis along center of IREP
%           stem and x axis pointing in the direction of parallelogram
%           opening
%       q_par=the corresponding q2, q3 values for the desired b1. 
%       L0=initial length of passive stem at home configuration. 
%       alpha is a compensation factor for accounting for the required pulling when the passive stem is commanded forward
%--------------------------------------------------------------------------
function [q1,q23]  = fcn(b1,q_par,L0)
%#eml
L = get_length_for_coordination([-b1(1);b1(2)]);
q_offset = L-L0;
% q1 = beta*q_offset; %insertion axis
q1 = q_offset; %insertion axis
% q23 = q_par - alpha*[q_offset;q_offset];
q23 = q_par - [q_offset;q_offset];

== matlab function Trajectory Planner/Right Arm/High Level/Configuration Space/Stem/5th Order Polynomial/Embedded MATLAB Function ==
  data: p_des input double; p_curr input double; tf input double; tc input double; p output double; pdot output double; conf input double; confn output double; t0 input double; t0n output double; p0n output double; p0 input double; enable input double
function [p,pdot,confn,t0n,p0n] = fifth_order_p(p_des,p_curr,tf,tc,conf,t0,p0,enable)

if enable == 0                  % Configuration space is not used (pdot = 0). 
    p = p_curr;          % However we do want to record the current 
    confn = 0;                  % position in order to be ready as soon 
    t0n = tc;                   % as the enable becomes 1. 
    p0n = p_curr;
    pdot = zeros(5,1);
else
    if (p_des-p0)'*(p_des-p0) > 0
        if conf == 0                % conf = 0 means that the 5th order poly 
            p0n = p0;               % is not configured for the desired trajectory.
            t0n = tc;               % Therefore, the block is initialized.
            confn = 1;
            p = p0;
            pdot = zeros(5,1);
        else
            p0n = p0;
            t0n = t0;
            confn = conf;
            % 5th order polynomial
            a0 = p0;
            a4 = -15*(p_des-p0);
            a3 = -2/3 * a4;
            a5 = -2/5 * a4;
            t = tc-t0;
            tau = t/tf;
            if t < tf
                p = a0 + a3 * tau^3 + a4 * tau^4 + a5 * tau^5;
                pdot = 3*a3*t^2/tf^3 + 4*a4*t^3/tf^4 + 5*a5*t^4/tf^5;
            else
                p = p_des;
                pdot = zeros(5,1);
                p0n = p_des;
            end
        end
    else
        p = p_des;
        pdot = zeros(5,1);
        confn = 0;
        p0n = p0;
        t0n = t0;
    end
end
%------------------------------------------------------------------------

== matlab function Trajectory Planner/UDP_SendTo_MTM/Right_UDP/pose_curr_scope/R_to_axis_angle2 ==
  data: R input double; n_vec output double; theta output double
function [n_vec,theta] = AxisAngle(R)
%#eml
% Axis_angle(R) gives the rotation axis and the rotation angle extracted from rotation matrix R
% Note this function handles singular cases even if theta=0 or theta=180
% degrees, which cause the normal axis equation to become undefined.
% Written by N. Simaan
% Last updated 10/14/2012.

cos_theta=(trace(R)-1)/2;
sin_theta=(1/2)*sqrt((R(3,2)-R(2,3))^2 + (R(1,3)-R(3,1))^2 + (R(2,1)-R(1,2))^2);
theta=atan2(sin_theta,cos_theta);
index=0;
if abs(sin_theta)>1e-6 % before it was 1e-12, Long Wang changed it.
    n_cross=1/(2*sin_theta)*(R-R');
    n_vec=[-n_cross(2,3);n_cross(1,3);-n_cross(1,2)]; %disp('aaa');
    n_vec=n_vec/norm(n_vec);
else
    if cos_theta>0  %this means identity matrix
        n_vec=[0;0;0]; %I choose this arbitrarily to designate the special case for identity matrix
    else  %this is the case where theta is 180 degrees
        nx=sqrt((R(1,1)-cos_theta)/(1-cos_theta));
        ny=sqrt((R(2,2)-cos_theta)/(1-cos_theta));
        nz=sqrt((R(3,3)-cos_theta)/(1-cos_theta));
        
        %%% find the axis that best fits the given rotation matrix
        signs=[[1;1;1],...
               [1;-1;1],...
               [1;-1;-1],...
               [1;1;-1],...
               [-1;1;1],...
               [-1;-1;1],...
               [-1;-1;-1],...
               [-1;1;-1]];
        
        e=zeros(1,8); 
        
        for i=1:1:8
            n_candidate=signs(:,i).*[nx;ny;nz];
            Temp=rotd(n_candidate,theta*180/pi), %rotd takes its input in degrees
            e(1,i)=sum(sum((Temp-R).*(Temp-R)));
        end;    
              e,
        e_min=min(e); %the best fit    
        index=0
        for i=1:1:8  %find the index of the combination that produces the closest rotation
            if e(1,i)==e_min 
                index=i;
                break; 
            end;
        end;
        
        n_vec=signs(:,index).*[nx;ny;nz];
    end
end

== matlab function Wrench Estimation/tau sensing compensation/friction compensation ==
  data: q_bb input double; tau_sensed input double; tau_comp output double; gain_tension input double; gain_compression input double; bias_tension input double; bias_compression input double; deadband input double
function tau_comp = fcn(q_bb,tau_sensed,gain_tension,gain_compression,bias_tension,bias_compression,deadband)
%#eml
% q_cur is 8x1
tau_comp = (q_bb>deadband).*gain_compression.*(tau_sensed - bias_compression) + ...
           (q_bb<-deadband).*gain_tension.*(tau_sensed - bias_tension) + ...
           (q_bb<=deadband).*(q_bb>=-deadband).*tau_sensed;
